simulink library "asbhl20env"  (R2016b)
settings: Solver=ode45  StartTime=0.0  StopTime=10.0  RelTol=1e-3
undefined symbols (not defined in the file): F, Light, mass, MIL
libraries: aerolibwind2 x3, aerolibconvert2 x2, aerolibatmos2 x1, aerolibgravity2 x1
Description:
  | HL-20 environment component module: atmosphere, wind, terrain (stub), gravity
settings Model: ExtModeAutoUpdateStatusClock=off  Creator=The MathWorks, Inc.  LastModifiedBy=The MathWorks, Inc.
settings DataIOCC: LimitDataPoints=on  SaveFormat=Array  SignalLoggingSaveFormat=ModelDataLogs
settings OptimizationCC: BlockReduction=off  BooleanDataType=off  ExpressionDepthLimit=2147483647  LifeSpan=inf
settings DebuggingCC: SaveWithParameterizedLinksMsg=none  UnderspecifiedInitializationDetection=Classic  MergeDetectMultiDrivingBlocksExec=none  SignalResolutionControl=TryResolveAllWithWarning  FcnCallInpInsideContextMsg=warning  AllowSymbolicDim=off  StateNameClashWarn=warning  StrictBusMsg=Warning  SFUnexpectedBacktrackingDiag=warning  SFNoUnconditionalDefaultTransitionDiag=warning  SFExecutionAtInitializationDiag=none
settings HardwareCC: ProdBitPerPointer=32  ProdBitPerSizeT=32  ProdBitPerPtrDiffT=32  ProdLargestAtomicFloat=None  ProdIntDivRoundTo=Undefined  ProdEndianess=Unspecified  ProdWordSize=32  ProdHWDeviceType=32-bit Generic  TargetUnknown=on
settings ModelReferenceCC: PropagateSignalLabelsOutOfModel=off
settings GRTTargetCC: TargetLangStandard=C89/C90 (ANSI)  GeneratePreprocessorConditionals=Disable all
settings ConfigComp: CovMetricSettings=dw  CovHtmlReporting=on  CovSaveCumulativeToWorkspaceVar=on  CovSaveSingleToWorkspaceVar=on  CovExternalEMLEnable=off

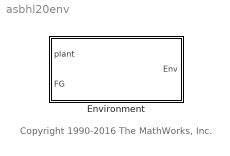
== system asbhl20env ==
  note: Copyright 1990-2016 The MathWorks, Inc.
  Environment : Subsystem  TreatAsAtomicUnit=on
      mask Display:
      | image('aeroenvironment.bmp','center')
      | port_label('input',1,'Env')
      | port_label('input',2,'FG')

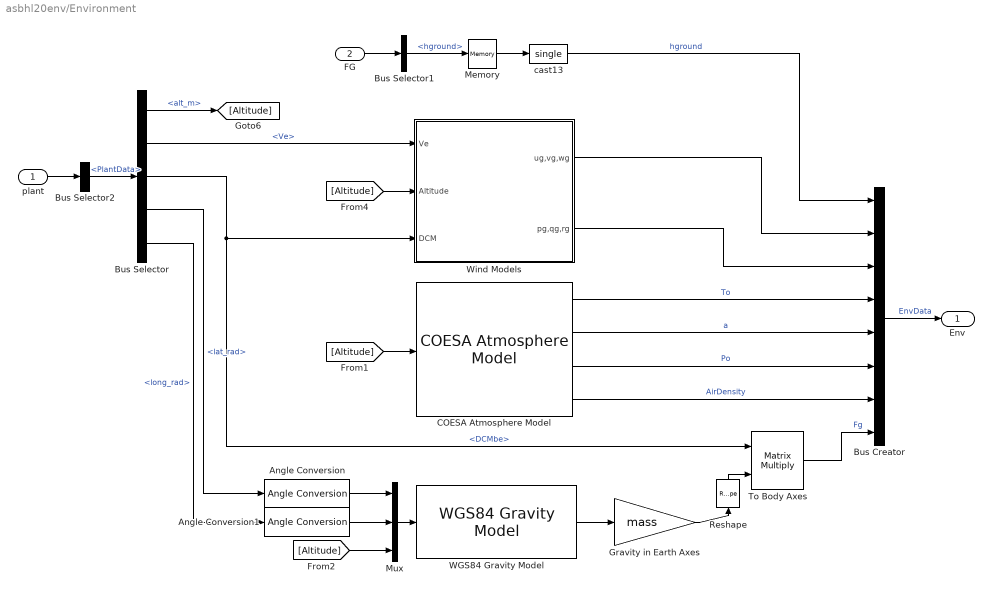
== system asbhl20env/Environment ==
  plant : Inport
  FG : Inport  Port=2  OutDataTypeStr=Bus: FlightGearBus
  Angle Conversion : aerolibconvert2/Angle Conversion  IU=rad  OU=deg
  Angle Conversion1 : aerolibconvert2/Angle Conversion  IU=rad  OU=deg
  Bus Creator : BusCreator  Inputs='hground','WindVelocity','WindAngularRates','To','a','Po','AirDensity','Fg'
  Bus Selector : BusSelector  OutputSignals=PosLLA.alt_m,Ve,DCMbe,PosLLA.lat_rad,PosLLA.long_rad
  Bus Selector1 : BusSelector  OutputSignals=hground
  Bus Selector2 : BusSelector  OutputSignals=PlantData
  COESA Atmosphere Model : aerolibatmos2/COESA Atmosphere Model  units=Metric (MKS)  spec=1976 COESA-extended U.S. Standard Atmosphere  model=Profile  profile_var=High temperature  profile_percent=1%  profile_alt=5 km (16404 ft)  envelope_var=High temperature  envelope_percent=1%  action=Warning
  Gravity in Earth Axes : Gain  Gain=mass  SaturateOnIntegerOverflow=on  OutDataTypeStr=Inherit: Same as input  ParamDataTypeStr=Inherit: Same as input
  Memory : Memory
  Mux : Mux  Inputs=3
  Reshape : Reshape
  To Body Axes : Product  Multiplication=Matrix(*)  SaturateOnIntegerOverflow=on  InputSameDT=on  OutDataTypeStr=Inherit: Same as first input
  "WGS84 Gravity Model " : aerolibgravity2/WGS84 Gravity Model   model=WGS84 Taylor Series  units=Metric (MKS)  no_atmos=on  precessing=on  jd_loc=off  month=October  day=10  year=2004  no_centrifugal=on  action=Warning
  Wind Models : Subsystem
  cast13 : DataTypeConversion  OutDataTypeStr=single  SaturateOnIntegerOverflow=on
  Env : Outport  InitialOutput=0
  wires:
  Reshape/1 -> To Body Axes/2
  Bus Selector1/1 -> Memory/1  "<hground>"
  Bus Selector2/1 -> Bus Selector/1  "<PlantData>"
  Wind Models/1(ug,vg,wg) -> Bus Creator/2
  Wind Models/2(pg,qg,rg) -> Bus Creator/3
  COESA Atmosphere Model/4 -> Bus Creator/7  "AirDensity"
  COESA Atmosphere Model/2 -> Bus Creator/5  "a"
  COESA Atmosphere Model/3 -> Bus Creator/6  "Po"
  COESA Atmosphere Model/1 -> Bus Creator/4  "To"
  Bus Selector/4 -> Angle Conversion/1  "<lat_rad>"
  "WGS84 Gravity Model "/1 -> Gravity in Earth Axes/1
  Gravity in Earth Axes/1 -> Reshape/1
  To Body Axes/1 -> Bus Creator/8  "Fg"
  Bus Creator/1 -> Env/1  "EnvData"
  plant/1 -> Bus Selector2/1
  Bus Selector/1 -> [Altitude]  "<alt_m>"
  [Altitude] -> Wind Models/2(Altitude)
  [Altitude] -> COESA Atmosphere Model/1
  Bus Selector/2 -> Wind Models/1(Ve)  "<Ve>"
  Bus Selector/3 -> Wind Models/3(DCM), To Body Axes/1  "<DCMbe>"
  Angle Conversion/1 -> Mux/1
  Bus Selector/5 -> Angle Conversion1/1  "<long_rad>"
  Mux/1 -> "WGS84 Gravity Model "/1
  Angle Conversion1/1 -> Mux/2
  [Altitude] -> Mux/3
  FG/1 -> Bus Selector1/1
  cast13/1 -> Bus Creator/1  "hground"
  Memory/1 -> cast13/1

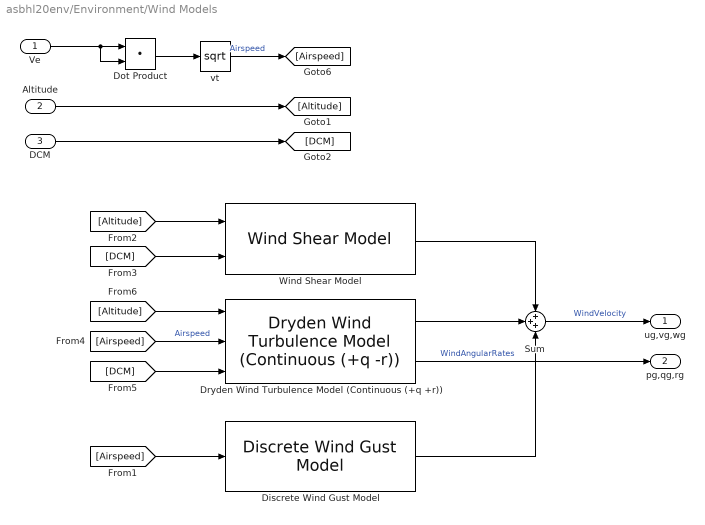
== system asbhl20env/Environment/Wind Models ==
  Ve : Inport
  Altitude : Inport  Port=2
  DCM : Inport  Port=3
  Discrete Wind Gust Model : aerolibwind2/Discrete Wind Gust Model  units=Metric (MKS)  Gx=on  Gy=on  Gz=on  t_0=20  d_m=[120 120 80]  v_m=[3.5 3.0 3.0]
  Dot Product : DotProduct  OutDataTypeStr=Inherit: Inherit via internal rule
  Dryden Wind Turbulence Model (Continuous (+q +r)) : aerolibwind2/Dryden Wind Turbulence Model  (Continuous (+q -r))  units=Metric (MKS)  spec=MIL-F-8785C  model=Continuous Dryden (+q +r)  W20=5  Wdeg=0  TurbProb=10^-2 - Light  L_high=533.4  Wingspan=4  ts=0.1  Seed=[23341 23342 23343 23344]  T_on=on
  Sum : Sum  Inputs=+++  SaturateOnIntegerOverflow=on  InputSameDT=on  OutDataTypeStr=Inherit: Same as first input
  Wind Shear Model : aerolibwind2/Wind Shear Model  units=Metric (MKS)  phase=Category C - Terminal Flight Phase  W_20=1  Wdeg=0
  vt : Math  Operator=sqrt  SaturateOnIntegerOverflow=on
  ug,vg,wg : Outport  Unit=m/s
  pg,qg,rg : Outport  Port=2  Unit=rad/s
  wires:
  Ve/1 -> Dot Product/1, Dot Product/2
  Wind Shear Model/1 -> Sum/1
  Dryden Wind Turbulence Model (Continuous (+q +r))/1 -> Sum/2
  Discrete Wind Gust Model/1 -> Sum/3
  Sum/1 -> ug,vg,wg/1  "WindVelocity"
  [Airspeed] -> Dryden Wind Turbulence Model (Continuous (+q +r))/2  "Airspeed"
  Dryden Wind Turbulence Model (Continuous (+q +r))/2 -> pg,qg,rg/1  "WindAngularRates"
  Dot Product/1 -> vt/1
  vt/1 -> [Airspeed]  "Airspeed"
  [Airspeed] -> Discrete Wind Gust Model/1
  Altitude/1 -> [Altitude]
  [Altitude] -> Wind Shear Model/1
  DCM/1 -> [DCM]
  [DCM] -> Wind Shear Model/2
  [DCM] -> Dryden Wind Turbulence Model (Continuous (+q +r))/3
  [Altitude] -> Dryden Wind Turbulence Model (Continuous (+q +r))/1
